simulink model "LACS"  (R2016b)
settings: Solver=VariableStepAuto  StartTime=0.0  StopTime=10  RelTol=1e-3
values from neighbouring files (symbols this model uses):
  coefficient = 0.8    [LACS.sldd]
  Detal_ref = 0.00022116955850615819 0.00022116955850615819 0.00024339323736781077 0.00026784369743330114 0.00029474273075037104 0.00032433393975435165 0.00035688482250496254 0.00039268904453642435 0.00043206891122917146 0.00047537805500027884 0.00052300435183202216 0.00057537308165349073 0.00063295034678974044 0.00069624676200566427 0.00076582142849131239 0.0008422862023284908 0.000926310265386283 0.0010186250    [LACS.sldd]    (also in path_generate.m = zeros(N,1))
  driver_decel = 4.0    [LACS.sldd]
  EgoLength = 3.048    [LACS.sldd]
  egopath = 0.0 0.25 0.5 0.75 1.0 1.25 1.5 1.7500000000000002 2.0 2.25 2.5 2.75 3.0 3.25 3.5000000000000004 3.75 4.0 4.25 4.5 4.75 5.0 5.25 5.5 5.75 6.0 6.25 6.5 6.75 7.0000000000000009 7.2499999999999991 7.5 7.75 8.0 8.25 8.5 8.75 9.0 9.25 9.5 9.75 10.0 10.25 10.5 10.75 11.0 11.25 11.5 11.75 12.0 12.25 12.5 12.75 13.0 13.25 13.5 13.750000000000002 14.000000000000002 14.250000000000002 14.499999999999998 14.7    [LACS.sldd]
  egoSpdLimit_H = 150.0    [LACS.sldd]
  egoSpdLimit_L = 10.0    [LACS.sldd]
  EgoWidth = 1.628    [LACS.sldd]
  ESA_Active = 3.0    [LACS.sldd]
  ESA_mask_1 = 31.0    [LACS.sldd]
  ESA_mask_2 = 15.0    [LACS.sldd]
  ESA_mask_3 = 255.0    [LACS.sldd]
  ESA_mask_4 = 31.0    [LACS.sldd]
  ESA_Passive = 1.0    [LACS.sldd]
  ESA_Standby = 2.0    [LACS.sldd]
  g = 9.8    [LACS.sldd]
  headwayoffset = 1.524    [LACS.sldd]
  LatAccelThershold = 0.05    [LACS.sldd]
  LatDis = 0.5    [LACS.sldd]
  LatSafetyThershold = 0.5    [LACS.sldd]
  LengthObj = 3.0    [LACS.sldd]
  ObjWidth = 2.0    [LACS.sldd]
  PB1_decel = 3.0    [LACS.sldd]
  PB2_decel = 5.0    [LACS.sldd]
  PB3_decel = 8.0    [LACS.sldd]
  Phi_dot_ref = 0.00085065224568106894 0.00085065224568106894 0.000936127966106986 0.0010301682404378703 0.0011336261186052523 0.0012474385378394444 0.001372634343205976 0.0015103430260158721 0.001661804233646022 0.0018283781058153412 0.0020115564932359636 0.0022129751145658549 0.0024344267064660809 0.0026778752189651235 0.0029454711038487576 0.0032395677369184911 0.0035627390050890382 0.0039177980756855638 0.004    [LACS.sldd]    (also in path_generate.m = zeros(N,1))
  Phi_ref = 0.00038406250525431664 0.00042271073336932769 0.00046524334565338114 0.00051204974395873044 0.000563558155980624 0.00062023946191088657 0.00068261138880285879 0.00075124310596315759 0.0008267602572639512 0.0009098504689462523 0.0010012693742370194 0.0011018471988988175 0.0012124959546271103 0.0013342172899504143 0.0014681110508986705 0.0016153846060911084 0.0017773629929370329 0.001955499943191484    [LACS.sldd]    (also in path_generate.m = phi_ref)
  SteerAngleLimit = 20.0    [LACS.sldd]
  SteerAngleSpdLimit = 20.0    [LACS.sldd]
  StrAngSpdThershold = 0.05    [LACS.sldd]
  StrAngThershold = 0.0    [LACS.sldd]
  Time2React = 1.2    [LACS.sldd]
  timeMargin = 0.5    [LACS.sldd]
  TTCthreshold1 = 2.5    [LACS.sldd]
  TTCthreshold3 = 1.0    [LACS.sldd]
  X_dot_ref = 10.0 10.0 10.0 9.9999999999999947 10.0 10.0 10.0 10.0 10.0 10.0 10.0 10.0 10.0 10.0 10.0 10.000000000000018 10.0 10.0 10.0 10.0 10.0 10.0 10.0 10.0 10.0 10.0 10.0 10.0 10.0 10.0 10.0 10.0 10.0 10.0 10.0 10.0 10.0 10.0 10.0 10.0 10.0 10.0 10.0 10.0 10.0 10.0 10.0 10.0 10.0 10.0 10.0 10.0 10.0 10.0 10.0 10.0 10.0 10.0 10.0 10.0 10.0 10.0 10.0 9.9999999999999289 10.0 10.0 10.0 10.0 10.0 10.0 10.0 10.    [LACS.sldd]    (also in path_generate.m = zeros(N,1))
  X_ref = 0.05 0.55 1.05 1.55 2.05 2.55 3.05 3.55 4.05 4.55 5.05 5.55 6.05 6.55 7.05 7.55 8.05 8.55 9.05 9.55 10.05 10.55 11.05 11.55 12.05 12.55 13.05 13.55 14.05 14.55 15.05 15.55 16.05 16.55 17.05 17.55 18.05 18.55 19.05 19.55 20.05 20.55 21.05 21.55 22.05 22.55 23.05 23.55 24.05 24.55 25.05 25.55 26.05 26.55 27.05 27.55 28.05 28.55 29.05 29.55 30.05 30.55 31.05 31.55 32.05 32.55 33.05 33.55 34.05 34.55    [LACS.sldd]    (also in path_generate.m = X_phi')
  Y_dot_ref = 0.0044363771042237217 0.0044363771042237217 0.00488273213335339 0.0053739322979981 0.0059144698111347933 0.0065092840662692251 0.0071638055584438178 0.0078840039934084845 0.0086764409570179273 0.0095483275445279979 0.01050758737719603 0.011562925461771293 0.012723903376023141 0.014001021290828194 0.015405807364013962 0.016950915064438028 0.018650229002128878 0.020518979854070446 0.0225738689793052    [LACS.sldd]    (also in path_generate.m = zeros(N,1))
  Y_ref = 0.0020016327462461514 0.0022031718511841521 0.0024249907063953382 0.0026691273130630077 0.0029378239279629127 0.0032335474185196523 0.0035590116218331136 0.0039172018997553045 0.0043114020994257287 0.0047452241472766251 0.005222640524503025 0.0057480198933628265 0.0063261661664513911 0.0069623613352525482 0.0076624123997939579 0.008432702767994656 0.0092802485212165574 0.010212759971323001 0.01123    [LACS.sldd]    (also in path_generate.m = zeros(N,1))
undefined symbols (not defined in the file or in its folder): ADR_ADRCycleTime, ADR_SteeringYawrateThresh_p, AEB_mask1, aubr, CAEB_AccelPdlPosLimit, CAEB_AccelPdlPosSpdThreshold, CAEB_CalAEBLongVelObjLimit_mps, CAEB_CalAEBVMaxDec_kmph, ESA_AESACTIVE, ESA_ERROR, ESA_ESAFunctionOFF, ESA_ESAFunctionON, ESA_ESASwichOFF, ESA_ESS_DriverSteeringNumThreshold, ESA_ESSACTIVE, ESA_ForewardCollissionLevel2, ESA_ForewardCollissionLevel3, ESA_OFF, ESA_PASSIVE, ESA_PLAN_AES, ESA_PLAN_ESSLEFT, ESA_PLAN_ESSRIGHT, ESA_PLAN_FAILURE, ESA_PLAN_OFF, ESA_PLAN_STANDBY, ESA_PLAN_WAIT, ESA_SPEEDLIMITH6_p, ESA_SPEEDLIMITH7_p, ESA_SPEEDLIMITL6_p, ESA_SPEEDLIMITL7_p, ESA_STANDBY, ESA_StrAngSpdT6_p, FromAngle2Rad, Kp, magnitude, tablebr, TTCthreshold, vubr
libraries: simulink x15, Solver_SF x9, simulink_extras x1
(part 2 of 5)

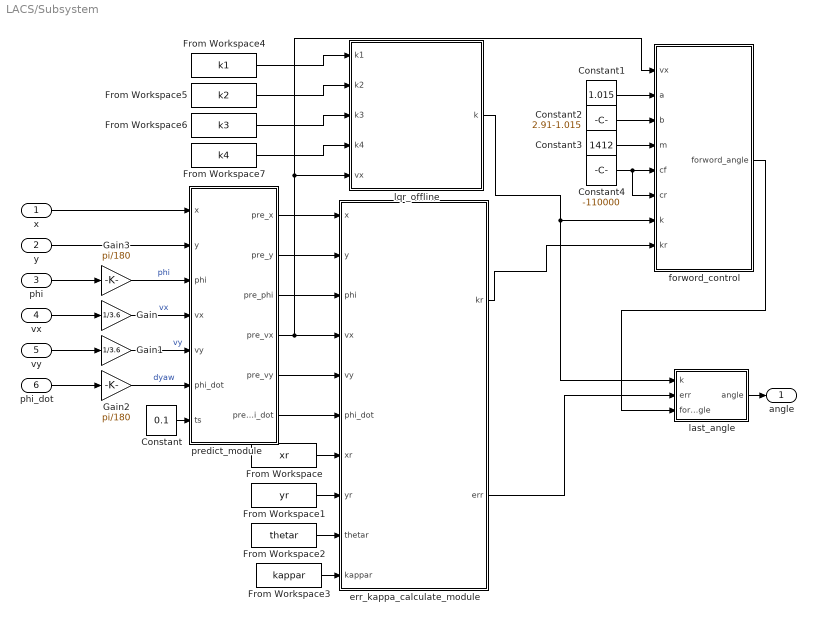
== system LACS/Subsystem ==
  x : Inport
  y : Inport  Port=2
  phi : Inport  Port=3
  vx : Inport  Port=4
  vy : Inport  Port=5
  phi_dot : Inport  Port=6
  Constant : Constant  Value=0.1
  Constant1 : Constant  Value=1.015
  Constant2 : Constant  Value=2.91-1.015
  Constant3 : Constant  Value=1412
  Constant4 : Constant  Value=-110000
  From Workspace : FromWorkspace  VariableName=xr  SampleTime=0
  From Workspace1 : FromWorkspace  VariableName=yr  SampleTime=0
  From Workspace2 : FromWorkspace  VariableName=thetar  SampleTime=0
  From Workspace3 : FromWorkspace  VariableName=kappar  SampleTime=0
  From Workspace4 : FromWorkspace  VariableName=k1  SampleTime=0
  From Workspace5 : FromWorkspace  VariableName=k2  SampleTime=0
  From Workspace6 : FromWorkspace  VariableName=k3  SampleTime=0
  From Workspace7 : FromWorkspace  VariableName=k4  SampleTime=0
  Gain : Gain  Gain=1/3.6
  Gain1 : Gain  Gain=1/3.6
  Gain2 : Gain  Gain=pi/180
  Gain3 : Gain  Gain=pi/180
  err_kappa_calculate_module : MATLAB Function  TreatAsAtomicUnit=on
  forword_control : MATLAB Function  TreatAsAtomicUnit=on
  last_angle : MATLAB Function  TreatAsAtomicUnit=on
  lqr_offline : MATLAB Function  TreatAsAtomicUnit=on
  predict_module : MATLAB Function  TreatAsAtomicUnit=on
  angle : Outport
  wires:
  From Workspace7/1 -> lqr_offline/4(k4)
  err_kappa_calculate_module/2(err) -> last_angle/2(err)
  Gain1/1 -> predict_module/5(vy)  "vy"
  From Workspace6/1 -> lqr_offline/3(k3)
  x/1 -> predict_module/1(x)
  lqr_offline/1(k) -> last_angle/1(k), forword_control/7(k)
  phi_dot/1 -> Gain2/1
  predict_module/2(pre_y) -> err_kappa_calculate_module/2(y)
  err_kappa_calculate_module/1(kr) -> forword_control/8(kr)
  forword_control/1(forword_angle) -> last_angle/3(forword_angle)
  vx/1 -> Gain/1
  predict_module/4(pre_vx) -> lqr_offline/5(vx), forword_control/1(vx), err_kappa_calculate_module/4(vx)
  Gain2/1 -> predict_module/6(phi_dot)  "dyaw"
  last_angle/1(angle) -> angle/1
  phi/1 -> Gain3/1
  From Workspace2/1 -> err_kappa_calculate_module/9(thetar)
  From Workspace5/1 -> lqr_offline/2(k2)
  Gain/1 -> predict_module/4(vx)  "vx"
  y/1 -> predict_module/2(y)
  Gain3/1 -> predict_module/3(phi)  "phi"
  From Workspace3/1 -> err_kappa_calculate_module/10(kappar)
  Constant/1 -> predict_module/7(ts)
  From Workspace4/1 -> lqr_offline/1(k1)
  From Workspace1/1 -> err_kappa_calculate_module/8(yr)
  predict_module/1(pre_x) -> err_kappa_calculate_module/1(x)
  predict_module/5(pre_vy) -> err_kappa_calculate_module/5(vy)
  vy/1 -> Gain1/1
  From Workspace/1 -> err_kappa_calculate_module/7(xr)
  predict_module/6(pre_phi_dot) -> err_kappa_calculate_module/6(phi_dot)
  predict_module/3(pre_phi) -> err_kappa_calculate_module/3(phi)
  Constant1/1 -> forword_control/2(a)
  Constant2/1 -> forword_control/3(b)
  Constant3/1 -> forword_control/4(m)
  Constant4/1 -> forword_control/6(cr), forword_control/5(cf)

== system LACS/TroqueOutput ==
  In1 : Inport
  Out1 : Outport

== system LACS/double_pid_controller ==
  s_dot : Inport
  v : Inport  Port=2
  es : Inport  Port=3
  rpm : Inport  Port=4
  vp : Inport  Port=5
  ap : Inport  Port=6
  Add : Sum  Inputs=-++
  Add2 : Sum
  Delay2 : Delay  DelayLength=1
  MATLAB Function1 : MATLAB Function  TreatAsAtomicUnit=on
  PID Controller : simulink/Continuous/PID Controller  Controller=PID  TimeDomain=Continuous-time  SampleTime=-1  IntegratorMethod=Forward Euler  FilterMethod=Forward Euler  Form=Parallel  UseFilter=on  ControllerParametersSource=internal  P=3  I=0  D=0.1  N=30  InitialConditionSource=internal  InitialConditionForIntegrator=0  InitialConditionForFilter=0  ExternalReset=none  LimitOutput=off  UpperSaturationLimit=inf  LowerSaturationLimit=-inf  LinearizeAsGain=on  AntiWindupMode=none  Kb=1  TrackingMode=off  Kt=1  PParamMin=[]  PParamMax=[]  IParamMin=[]  IParamMax=[]  DParamMin=[]  DParamMax=[]  NParamMin=[]  NParamMax=[]  KbParamMin=[]  KbParamMax=[]  KtParamMin=[]  KtParamMax=[]  POutMin=[]  POutMax=[]  IOutMin=[]  IOutMax=[]  DOutMin=[]  DOutMax=[]  NOutMin=[]  NOutMax=[]  KbOutMin=[]  KbOutMax=[]  KtOutMin=[]  KtOutMax=[]  IntegratorOutMin=[]  IntegratorOutMax=[]  FilterOutMin=[]  FilterOutMax=[]  SumOutMin=[]  SumOutMax=[]  SumI1OutMin=[]  SumI1OutMax=[]  SumI2OutMin=[]  SumI2OutMax=[]  SumI3OutMin=[]  SumI3OutMax=[]  SumDOutMin=[]  SumDOutMax=[]  SaturationOutMin=[]  SaturationOutMax=[]  IntegratorContinuousStateAttributes=''  IntegratorStateMustResolveToSignalObject=off  IntegratorRTWStateStorageClass=Auto  FilterContinuousStateAttributes=''  FilterStateMustResolveToSignalObject=off  FilterRTWStateStorageClass=Auto  DifferentiatorICPrevScaledInput=0  DifferentiatorOutMin=[]  DifferentiatorOutMax=[]
  PID Controller1 : simulink/Continuous/PID Controller  Controller=PID  TimeDomain=Continuous-time  SampleTime=-1  IntegratorMethod=Forward Euler  FilterMethod=Forward Euler  Form=Parallel  UseFilter=on  ControllerParametersSource=internal  P=3  I=0  D=0.1  N=30  InitialConditionSource=internal  InitialConditionForIntegrator=0  InitialConditionForFilter=0  ExternalReset=none  LimitOutput=off  UpperSaturationLimit=inf  LowerSaturationLimit=-inf  LinearizeAsGain=on  AntiWindupMode=none  Kb=1  TrackingMode=off  Kt=1  PParamMin=[]  PParamMax=[]  IParamMin=[]  IParamMax=[]  DParamMin=[]  DParamMax=[]  NParamMin=[]  NParamMax=[]  KbParamMin=[]  KbParamMax=[]  KtParamMin=[]  KtParamMax=[]  POutMin=[]  POutMax=[]  IOutMin=[]  IOutMax=[]  DOutMin=[]  DOutMax=[]  NOutMin=[]  NOutMax=[]  KbOutMin=[]  KbOutMax=[]  KtOutMin=[]  KtOutMax=[]  IntegratorOutMin=[]  IntegratorOutMax=[]  FilterOutMin=[]  FilterOutMax=[]  SumOutMin=[]  SumOutMax=[]  SumI1OutMin=[]  SumI1OutMax=[]  SumI2OutMin=[]  SumI2OutMax=[]  SumI3OutMin=[]  SumI3OutMax=[]  SumDOutMin=[]  SumDOutMax=[]  SaturationOutMin=[]  SaturationOutMax=[]  IntegratorContinuousStateAttributes=''  IntegratorStateMustResolveToSignalObject=off  IntegratorRTWStateStorageClass=Auto  FilterContinuousStateAttributes=''  FilterStateMustResolveToSignalObject=off  FilterRTWStateStorageClass=Auto  DifferentiatorICPrevScaledInput=0  DifferentiatorOutMin=[]  DifferentiatorOutMax=[]
  Saturation : Saturate  UpperLimit=5  LowerLimit=-8
  Saturation1 : Saturate  UpperLimit=10  LowerLimit=-10
  moto model : MATLAB Function  TreatAsAtomicUnit=on
  油门刹车合并标定表 : Lookup_n-D  BreakpointsForDimension1=vubr  BreakpointsForDimension2=aubr  Table=tablebr  InternalRulePriority=Speed  RndMeth=Simplest  InputSameDT=on
  Out1 : Outport
  Out2 : Outport  Port=2
  wires:
  v/1 -> Delay2/1
  ap/1 -> Add2/2
  Add2/1 -> Saturation/1
  Saturation/1 -> 油门刹车合并标定表/2
  Delay2/1 -> 油门刹车合并标定表/1
  油门刹车合并标定表/1 -> MATLAB Function1/1(x)
  Add/1 -> PID Controller/1
  PID Controller/1 -> Add2/1
  MATLAB Function1/1(thr) -> moto model/1(thr)
  PID Controller1/1 -> Saturation1/1
  moto model/1(torque) -> Out1/1
  MATLAB Function1/2(brake) -> Out2/1
  vp/1 -> Add/3
  es/1 -> PID Controller1/1
  s_dot/1 -> Add/1
  rpm/1 -> moto model/2(rpm)
  Saturation1/1 -> Add/2

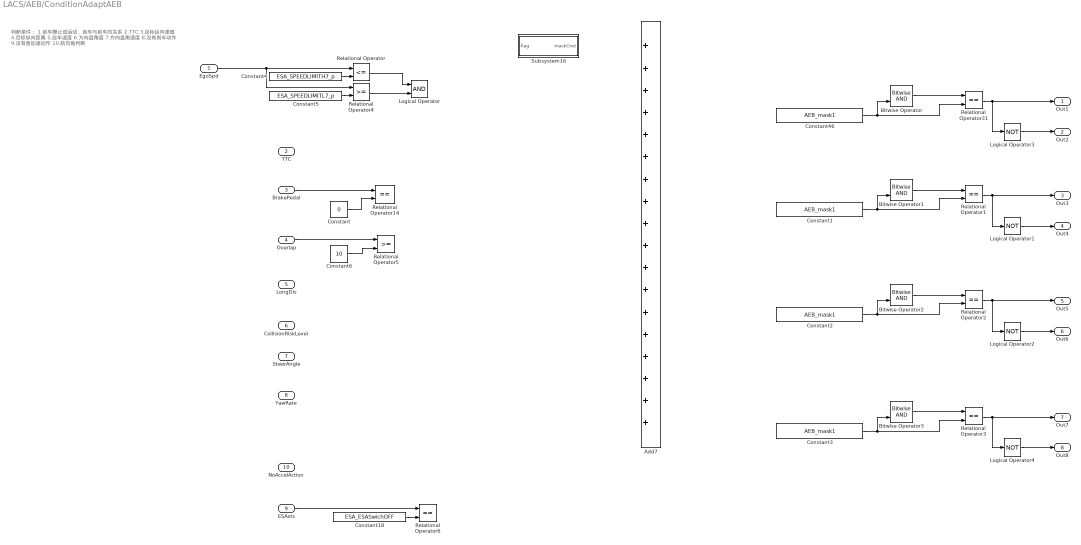
== system LACS/AEB/ConditionAdaptAEB ==
  note: 判断条件：
      | 1.前车静止或运动，自车与前车的关系
      | 2.TTC
      | 3.目标纵向速度
      | 4.目标纵向距离
      | 5.自车速度
      | 6.方向盘角度
      | 7.方向盘角速度
      | 8.没有刹车动作
      | 9.没有急加速动作
      | 10.航向角判断
  EgoSpd : Inport
  TTC : Inport  Port=2
  BrakePedal : Inport  Port=3
  Overlap : Inport  Port=4
  LongDis : Inport  Port=5
  CollisionRiskLevel : Inport  Port=6
  SteerAngle : Inport  Port=7
  YawRate : Inport  Port=8
  ESAsts : Inport  Port=9
  NoAccelAction : Inport  Port=10
  Add7 : Sum  Inputs=18  SaturateOnIntegerOverflow=on
  Bitwise Operator{,1..3} (4 alike) : simulink/Logic and Bit Operations/Bitwise Operator  logicop=AND  UseBitMask=off  NumInputPorts=2  BitMask=bin2dec('11011001')  BitMaskRealWorld=Stored Integer
  Constant : Constant  Value=0
  Constant{1..3,46} (4 alike) : Constant  Value=AEB_mask1  OutDataTypeStr=uint32
  Constant18 : Constant  Value=ESA_ESASwichOFF
  Constant4 : Constant  Value=ESA_SPEEDLIMITH7_p
  Constant5 : Constant  Value=ESA_SPEEDLIMITL7_p
  Constant6 : Constant  Value=10
  Logical Operator : Logic  AllPortsSameDT=off  OutDataTypeStr=boolean
  Logical Operator{1..4} (4 alike) : Logic  Operator=NOT  AllPortsSameDT=off  OutDataTypeStr=boolean
  Relational Operator : RelationalOperator  Operator=<=  OutDataTypeStr=boolean  RndMeth=Simplest
  Relational Operator{1..3,6,14,31} (6 alike) : RelationalOperator  Operator===  OutDataTypeStr=boolean  RndMeth=Simplest
  Relational Operator4 : RelationalOperator  OutDataTypeStr=boolean  RndMeth=Simplest
  Relational Operator5 : RelationalOperator  OutDataTypeStr=boolean  RndMeth=Simplest
  Subsystem16 : Subsystem
  Out1 : Outport
  Out2 : Outport  Port=2
  Out3 : Outport  Port=3
  Out4 : Outport  Port=4
  Out5 : Outport  Port=5
  Out6 : Outport  Port=6
  Out7 : Outport  Port=7
  Out8 : Outport  Port=8
  wires:
  Constant46/1 -> Bitwise Operator/2, Relational Operator31/2
  Bitwise Operator/1 -> Relational Operator31/1
  Relational Operator31/1 -> Logical Operator3/1, Out1/1
  Logical Operator3/1 -> Out2/1
  Constant1/1 -> Bitwise Operator1/2, Relational Operator1/2
  Bitwise Operator1/1 -> Relational Operator1/1
  Relational Operator1/1 -> Logical Operator1/1, Out3/1
  Logical Operator1/1 -> Out4/1
  Constant2/1 -> Bitwise Operator2/2, Relational Operator2/2
  Bitwise Operator2/1 -> Relational Operator2/1
  Relational Operator2/1 -> Logical Operator2/1, Out5/1
  Logical Operator2/1 -> Out6/1
  Constant3/1 -> Bitwise Operator3/2, Relational Operator3/2
  Bitwise Operator3/1 -> Relational Operator3/1
  Relational Operator3/1 -> Logical Operator4/1, Out7/1
  Logical Operator4/1 -> Out8/1
  Constant/1 -> Relational Operator14/2
  BrakePedal/1 -> Relational Operator14/1
  Relational Operator/1 -> Logical Operator/1
  Relational Operator4/1 -> Logical Operator/2
  EgoSpd/1 -> Relational Operator/1, Relational Operator4/1
  Constant4/1 -> Relational Operator/2
  Constant5/1 -> Relational Operator4/2
  Constant6/1 -> Relational Operator5/2
  Overlap/1 -> Relational Operator5/1
  ESAsts/1 -> Relational Operator6/1
  Constant18/1 -> Relational Operator6/2

== system LACS/AEB/DrvRapidAccelAction ==
  AccelPedalPos : Inport
  Add : Sum  Inputs=+-
  CAEB_AccelPdlPosLimit : Constant  Value=CAEB_AccelPdlPosLimit  OutDataTypeStr=Inherit: Inherit via back propagation
  CAEB_IPBInputRodStrokeSpdThreshold : Constant  Value=CAEB_AccelPdlPosSpdThreshold  OutDataTypeStr=single
  Constant4 : Constant  Value=0.02  OutDataTypeStr=single
  Data Type Conversion : DataTypeConversion
  Delay : Delay  DelayLength=1
  Divide : Product  Inputs=*//
  Logical Operator : Logic  AllPortsSameDT=off  OutDataTypeStr=boolean
  Relational Operator17 : RelationalOperator  OutDataTypeStr=boolean  RndMeth=Simplest
  Relational Operator4 : RelationalOperator  OutDataTypeStr=boolean  RndMeth=Simplest
  Saturation : Saturate  UpperLimit=inf  LowerLimit=0.0001
  DrvRapidAccelAction : Outport
  wires:
  CAEB_AccelPdlPosLimit/1 -> Relational Operator17/2
  Delay/1 -> Add/2
  Add/1 -> Divide/1
  AccelPedalPos/1 -> Data Type Conversion/1, Delay/1, Add/1, Relational Operator17/1
  Data Type Conversion/1 -> Saturation/1
  Saturation/1 -> Divide/2
  Constant4/1 -> Divide/3
  Divide/1 -> Relational Operator4/1
  CAEB_IPBInputRodStrokeSpdThreshold/1 -> Relational Operator4/2
  Relational Operator17/1 -> Logical Operator/1
  Relational Operator4/1 -> Logical Operator/2
  Logical Operator/1 -> DrvRapidAccelAction/1

== system LACS/AEB/TTCCaculation ==
  LongiVel : Inport
  LongiDis : Inport  Port=2
  Abs : Abs
  Abs1 : Abs
  Divide : Product  Inputs=*/
  Saturation1 : Saturate  UpperLimit=inf  LowerLimit=CAEB_CalAEBLongVelObjLimit_mps
  Saturation2 : Saturate  UpperLimit=inf  LowerLimit=CAEB_CalAEBLongVelObjLimit_mps
  TTC : Outport
  wires:
  LongiVel/1 -> Abs/1
  Abs/1 -> Saturation1/1
  LongiDis/1 -> Saturation2/1
  Abs1/1 -> TTC/1
  Divide/1 -> Abs1/1
  Saturation2/1 -> Divide/1
  Saturation1/1 -> Divide/2

== system LACS/AEB//ESAModeSwitch/If Action Subsystem ==
  Action Port : ActionPort  ActionType=then
  Constant1 : Constant  OutDataTypeStr=boolean
  Constant2 : Constant  Value=0  OutDataTypeStr=boolean
  ESAVTakeOverReq : Outport
  AEBVCrashAvoid : Outport  Port=2
  wires:
  Constant1/1 -> ESAVTakeOverReq/1
  Constant2/1 -> AEBVCrashAvoid/1

== system LACS/AEB//ESAModeSwitch/If Action Subsystem1 ==
  AEBTTCVaild : Inport
  EgoSpd : Inport  Port=2
  AEBTTC : Inport  Port=3
  Action Port : ActionPort  ActionType=else
  If : If  IfExpression=u1==0|u1==1|u1==4  ElseIfExpressions=u1==2
  If Action Subsystem : Subsystem  TreatAsAtomicUnit=on
  If Action Subsystem1 : Subsystem  TreatAsAtomicUnit=on
  If Action Subsystem2 : Subsystem  TreatAsAtomicUnit=on
  Merge : Merge  Inputs=3
  Merge1 : Merge  Inputs=3
  ESAVTakeOverReq : Outport
  AEBVCrashAvoid : Outport  Port=2
  wires:
  If/1 -> If Action Subsystem/Action
  If/2 -> If Action Subsystem1/Action
  If/3 -> If Action Subsystem2/Action
  Merge/1 -> ESAVTakeOverReq/1
  If Action Subsystem/1(ESAVTakeOverReq) -> Merge/1
  If Action Subsystem1/1(ESAVTakeOverReq) -> Merge/2
  If Action Subsystem2/1(ESAVTakeOverReq) -> Merge/3
  If Action Subsystem1/2(AEBVCrashAvoid) -> Merge1/2
  Merge1/1 -> AEBVCrashAvoid/1
  If Action Subsystem/2(AEBVCrashAvoid) -> Merge1/1
  If Action Subsystem2/2(AEBVCrashAvoid) -> Merge1/3
  AEBTTCVaild/1 -> If Action Subsystem/1(AEBTTCVaild), If/1
  AEBTTC/1 -> If Action Subsystem/2(AEBTTC), If Action Subsystem1/1(AEBTTC)
  EgoSpd/1 -> If Action Subsystem/3(EgoSpd), If Action Subsystem1/2(EgoSpd)

== system LACS/AEB//ESAModeSwitch/Subsystem ==
  SteerAngle : Inport
  SteerAngleSpd : Inport  Port=2
  Abs : Abs
  Abs1 : Abs
  Add1 : Sum  SaturateOnIntegerOverflow=on
  Add3 : Sum  SaturateOnIntegerOverflow=on
  Constant1 : Constant  Value=ESA_SPEEDLIMITH6_p
  Constant17 : Constant  OutDataTypeStr=uint8
  Constant18 : Constant  Value=0  OutDataTypeStr=uint8
  Constant2 : Constant  Value=ESA_SPEEDLIMITH6_p
  Constant22 : Constant  Value=ESA_StrAngSpdT6_p
  Constant3 : Constant  OutDataTypeStr=uint8
  Constant4 : Constant  Value=0  OutDataTypeStr=uint8
  Constant5 : Constant  Value=ESA_StrAngSpdT6_p
  Logical Operator : Logic  AllPortsSameDT=off  OutDataTypeStr=boolean
  Multiport Switch1 : MultiPortSwitch  DataPortOrder=Zero-based contiguous  Inputs=2
  Multiport Switch2 : MultiPortSwitch  DataPortOrder=Zero-based contiguous  Inputs=2
  Relational Operator{1..3,19} (4 alike) : RelationalOperator  OutDataTypeStr=boolean  RndMeth=Simplest
  Unit Delay1 : UnitDelay  SampleTime=-1
  Unit Delay2 : UnitDelay  SampleTime=-1
  DrvRapidSteerAction : Outport
  wires:
  Abs/1 -> Relational Operator2/1
  Relational Operator19/1 -> Logical Operator/1
  Constant1/1 -> Relational Operator1/2
  Abs1/1 -> Relational Operator1/1
  SteerAngleSpd/1 -> Abs1/1
  Logical Operator/1 -> DrvRapidSteerAction/1
  Multiport Switch2/1 -> Relational Operator19/1, Unit Delay2/1
  Constant2/1 -> Relational Operator2/2
  SteerAngle/1 -> Abs/1
  Constant18/1 -> Multiport Switch2/2
  Relational Operator2/1 -> Multiport Switch2/1
  Add3/1 -> Multiport Switch2/3
  Constant22/1 -> Relational Operator19/2
  Constant17/1 -> Add3/1
  Unit Delay2/1 -> Add3/2
  Relational Operator3/1 -> Logical Operator/2
  Constant4/1 -> Multiport Switch1/2
  Relational Operator1/1 -> Multiport Switch1/1
  Constant3/1 -> Add1/1
  Add1/1 -> Multiport Switch1/3
  Unit Delay1/1 -> Add1/2
  Constant5/1 -> Relational Operator3/2
  Multiport Switch1/1 -> Relational Operator3/1, Unit Delay1/1

== system LACS/AEBsts/Brake2StopTime ==
  EgoSpd : Inport
  CMpa1 : Inport  Port=2
  CMpa2 : Inport  Port=3
  CMpa3 : Inport  Port=4
  Add{1..4} (4 alike) : Sum
  Constant : Constant  Value=driver_decel
  Constant1 : Constant  Value=timeMargin
  Constant2 : Constant  Value=Time2React
  Divide{,1..3} (4 alike) : Product  Inputs=*/
  FCWStoppingTime : Outport
  PB1StoppingTime : Outport  Port=2
  PB2StoppingTime : Outport  Port=3
  FBStoppingTime : Outport  Port=4
  tag scope: FBStoppingTime=global, FCWStopTime_M=global, PB1StoppingTime_M=global, PB2StoppingTime_M=global
  wires:
  Constant/1 -> Divide/2
  EgoSpd/1 -> Divide1/1, Divide3/1, Divide2/1, Divide/1
  Constant2/1 -> Add1/1
  Divide/1 -> Add1/2
  Add1/1 -> [FCWStopTime_M], FCWStoppingTime/1
  Constant1/1 -> Add4/1, Add3/1, Add2/1
  Divide1/1 -> Add2/2
  CMpa2/1 -> Divide2/2
  Divide2/1 -> Add3/2
  Add3/1 -> [PB2StoppingTime_M], PB2StoppingTime/1
  CMpa3/1 -> Divide3/2
  Divide3/1 -> Add4/2
  Add4/1 -> [FBStoppingTime], FBStoppingTime/1
  Add2/1 -> [PB1StoppingTime_M], PB1StoppingTime/1
  CMpa1/1 -> Divide1/2

== system LACS/AEBsts/TTCCaculation ==
  LongiDis : Inport
  LongiVel : Inport  Port=2
  Abs : Abs
  Abs1 : Abs
  Add : Sum  Inputs=+-
  Constant : Constant  Value=headwayoffset
  Constant1 : Constant  Value=0.1
  Divide : Product  Inputs=*/
  Relational Operator4 : RelationalOperator  Operator=<  OutDataTypeStr=boolean  RndMeth=Simplest
  collision : Outport
  TTC : Outport  Port=2
  tag scope: LongiDis_M=global, Longivel_M=global, TTC_M=global, collision_M=global
  wires:
  LongiVel/1 -> Abs/1
  Abs/1 -> [Longivel_M], Divide/2
  LongiDis/1 -> [LongiDis_M], Add/1
  Add/1 -> Relational Operator4/1, Divide/1
  Constant/1 -> Add/2
  Constant1/1 -> Relational Operator4/2
  Relational Operator4/1 -> [collision_M], collision/1
  Divide/1 -> Abs1/1
  Abs1/1 -> [TTC_M], TTC/1

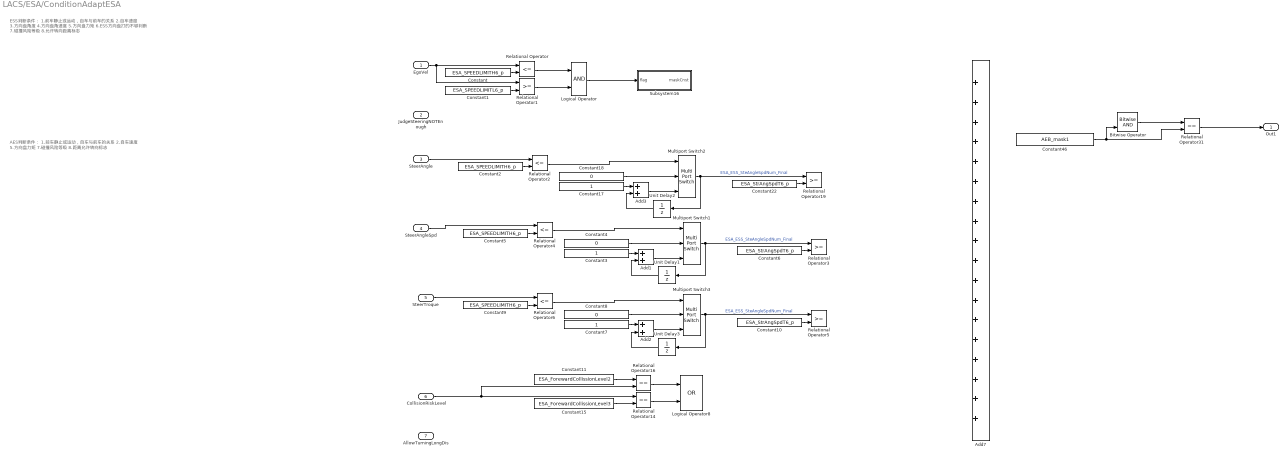
== system LACS/ESA/ConditionAdaptESA ==
  note: ESS判断条件：
      | 1.前车静止或运动，自车与前车的关系
      | 2.自车速度
      | 3.方向盘角度
      | 4.方向盘角速度
      | 5.方向盘力矩
      | 6.ESS方向盘打的不够判断
      | 7.碰撞风险等级
      | 8.允许转向距离标志
  note: AES判断条件：
      | 1.前车静止或运动，自车与前车的关系
      | 2.自车速度
      | 5.方向盘力矩
      | 7.碰撞风险等级
      | 8.距离允许转向标志
  EgoVel : Inport
  JudgeSteeringNOTEnough : Inport  Port=2
  SteerAngle : Inport  Port=3
  SteerAngleSpd : Inport  Port=4
  SteerTroque : Inport  Port=5
  CollisionRiskLevel : Inport  Port=6
  AllowTurningLongDis : Inport  Port=7
  Add1 : Sum  SaturateOnIntegerOverflow=on
  Add2 : Sum  SaturateOnIntegerOverflow=on
  Add3 : Sum  SaturateOnIntegerOverflow=on
  Add7 : Sum  Inputs=18  SaturateOnIntegerOverflow=on
  Bitwise Operator : simulink/Logic and Bit Operations/Bitwise Operator  logicop=AND  UseBitMask=off  NumInputPorts=2  BitMask=bin2dec('11011001')  BitMaskRealWorld=Stored Integer
  Constant{,2,5,9} (4 alike) : Constant  Value=ESA_SPEEDLIMITH6_p
  Constant1 : Constant  Value=ESA_SPEEDLIMITL6_p
  Constant10 : Constant  Value=ESA_StrAngSpdT6_p
  Constant11 : Constant  Value=ESA_ForewardCollissionLevel2  OutDataTypeStr=uint8
  Constant15 : Constant  Value=ESA_ForewardCollissionLevel3  OutDataTypeStr=uint8
  Constant17 : Constant  OutDataTypeStr=uint8
  Constant18 : Constant  Value=0  OutDataTypeStr=uint8
  Constant22 : Constant  Value=ESA_StrAngSpdT6_p
  Constant3 : Constant  OutDataTypeStr=uint8
  Constant4 : Constant  Value=0  OutDataTypeStr=uint8
  Constant46 : Constant  Value=AEB_mask1  OutDataTypeStr=uint32
  Constant6 : Constant  Value=ESA_StrAngSpdT6_p
  Constant7 : Constant  OutDataTypeStr=uint8
  Constant8 : Constant  Value=0  OutDataTypeStr=uint8
  Logical Operator : Logic  AllPortsSameDT=off  OutDataTypeStr=boolean
  Logical Operator8 : Logic  Operator=OR  AllPortsSameDT=off  OutDataTypeStr=boolean
  Multiport Switch1 : MultiPortSwitch  DataPortOrder=Zero-based contiguous  Inputs=2
  Multiport Switch2 : MultiPortSwitch  DataPortOrder=Zero-based contiguous  Inputs=2
  Multiport Switch3 : MultiPortSwitch  DataPortOrder=Zero-based contiguous  Inputs=2
  Relational Operator{,2,4,6} (4 alike) : RelationalOperator  Operator=<=  OutDataTypeStr=boolean  RndMeth=Simplest
  Relational Operator{1,3,5,19} (4 alike) : RelationalOperator  OutDataTypeStr=boolean  RndMeth=Simplest
  Relational Operator14 : RelationalOperator  Operator===  OutDataTypeStr=boolean  RndMeth=Simplest
  Relational Operator16 : RelationalOperator  Operator===  OutDataTypeStr=boolean  RndMeth=Simplest
  Relational Operator31 : RelationalOperator  Operator===  OutDataTypeStr=boolean  RndMeth=Simplest
  Subsystem16 : Subsystem
  Unit Delay1 : UnitDelay  SampleTime=-1
  Unit Delay2 : UnitDelay  SampleTime=-1
  Unit Delay3 : UnitDelay  SampleTime=-1
  Out1 : Outport
  wires:
  Constant46/1 -> Bitwise Operator/2, Relational Operator31/2
  Bitwise Operator/1 -> Relational Operator31/1
  Relational Operator31/1 -> Out1/1
  Constant1/1 -> Relational Operator1/2
  Constant/1 -> Relational Operator/2
  EgoVel/1 -> Relational Operator/1, Relational Operator1/1
  Relational Operator1/1 -> Logical Operator/2
  Relational Operator/1 -> Logical Operator/1
  Logical Operator/1 -> Subsystem16/1(flag)
  Constant2/1 -> Relational Operator2/2
  SteerAngle/1 -> Relational Operator2/1
  Add3/1 -> Multiport Switch2/3
  Constant17/1 -> Add3/1
  Unit Delay2/1 -> Add3/2
  Constant22/1 -> Relational Operator19/2
  Multiport Switch2/1 -> Unit Delay2/1, Relational Operator19/1  "ESA_ESS_SteAngleSpdNum_Final"
  Constant18/1 -> Multiport Switch2/2
  Relational Operator2/1 -> Multiport Switch2/1
  Constant5/1 -> Relational Operator4/2
  SteerAngleSpd/1 -> Relational Operator4/1
  Add1/1 -> Multiport Switch1/3
  Constant3/1 -> Add1/1
  Unit Delay1/1 -> Add1/2
  Constant6/1 -> Relational Operator3/2
  Multiport Switch1/1 -> Unit Delay1/1, Relational Operator3/1  "ESA_ESS_SteAngleSpdNum_Final"
  Constant4/1 -> Multiport Switch1/2
  Relational Operator4/1 -> Multiport Switch1/1
  Constant9/1 -> Relational Operator6/2
  SteerTroque/1 -> Relational Operator6/1
  Add2/1 -> Multiport Switch3/3
  Constant7/1 -> Add2/1
  Unit Delay3/1 -> Add2/2
  Constant10/1 -> Relational Operator5/2
  Multiport Switch3/1 -> Unit Delay3/1, Relational Operator5/1  "ESA_ESS_SteAngleSpdNum_Final"
  Constant8/1 -> Multiport Switch3/2
  Relational Operator6/1 -> Multiport Switch3/1
  Constant15/1 -> Relational Operator14/2
  CollisionRiskLevel/1 -> Relational Operator16/2, Relational Operator14/1
  Constant11/1 -> Relational Operator16/1
  Relational Operator16/1 -> Logical Operator8/1
  Relational Operator14/1 -> Logical Operator8/2

== system LACS/ESA/Control ==
  In1 : Inport
  Out1 : Outport

== system LACS/ESA/OverlapCaculation ==
  LatSpd : Inport
  TTC : Inport  Port=2
  LatDis : Inport  Port=3
  VehicleWidth : Inport  Port=4
  Abs : Abs
  Add5 : Sum
  Add6 : Sum  Inputs=+-
  Constant1 : Constant  Value=100
  Constant2 : Constant  Value=100
  Constant3 : Constant  Value=0.5
  Divide : Product  Inputs=*/
  Product1 : Product
  Product2 : Product
  Product3 : Product
  Saturation1 : Saturate  UpperLimit=20  LowerLimit=-20
  Saturation2 : Saturate  UpperLimit=100  LowerLimit=0
  OverLap : Outport
  wires:
  LatSpd/1 -> Product1/1
  TTC/1 -> Product1/2
  Constant2/1 -> Product2/1
  Divide/1 -> Product2/2
  VehicleWidth/1 -> Product3/1
  Saturation2/1 -> Add6/2
  Constant1/1 -> Add6/1
  LatDis/1 -> Add5/2
  Add6/1 -> OverLap/1
  Add5/1 -> Saturation1/1
  Product1/1 -> Add5/1
  Product2/1 -> Saturation2/1
  Product3/1 -> Divide/2
  Constant3/1 -> Product3/2
  Abs/1 -> Divide/1
  Saturation1/1 -> Abs/1

== system LACS/ESA/SteerDirection ==
  note: ESAsts=ESS
  ESAsts : Inport
  YawRate : Inport  Port=2
  FixSelectObs : Inport  Port=3
  Constant : Constant  Value=0
  Constant1 : Constant  Value=0
  If : If  IfExpression=u1 == 3  ElseIfExpressions=u1 == 4
  If Action Subsystem1 : Subsystem  TreatAsAtomicUnit=on
  Logical Operator : Logic  AllPortsSameDT=off  OutDataTypeStr=boolean
  Logical Operator1 : Logic  AllPortsSameDT=off  OutDataTypeStr=boolean
  Relational Operator : RelationalOperator  Operator=>  OutDataTypeStr=boolean  RndMeth=Simplest
  Relational Operator1 : RelationalOperator  Operator=<  OutDataTypeStr=boolean  RndMeth=Simplest
  Subsystem : Subsystem
  Subsystem1 : Subsystem
  ESS_LeftCtrl : Outport
  ESS_RightCtrl : Outport  Port=2
  CtrlInvaild : Outport  Port=3
  AES_LeftCtrl : Outport  Port=4
  AES_RightCtrl : Outport  Port=5
  wires:
  ESAsts/1 -> If/1
  If/1 -> Subsystem/Action
  If/3 -> If Action Subsystem1/Action
  Subsystem/1(Out2) -> Logical Operator1/1, Logical Operator/1
  Constant/1 -> Relational Operator/2
  Relational Operator/1 -> Logical Operator/2
  YawRate/1 -> Relational Operator1/1, Relational Operator/1, Subsystem/1(In1)
  Constant1/1 -> Relational Operator1/2
  Relational Operator1/1 -> Logical Operator1/2
  If Action Subsystem1/1(Out1) -> CtrlInvaild/1
  Logical Operator/1 -> ESS_LeftCtrl/1
  Logical Operator1/1 -> ESS_RightCtrl/1
  If/2 -> Subsystem1/Action
  FixSelectObs/1 -> Subsystem1/1(In1)
  Subsystem1/1(Left) -> AES_LeftCtrl/1
  Subsystem1/2(Right) -> AES_RightCtrl/1

== system LACS/ESA/TrajactoryPlan ==
  EgoSpd : Inport
  YawRate : Inport  Port=2
  Abs : Abs
  Constant : Constant  Value=ADR_SteeringYawrateThresh_p  OutDataTypeStr=single
  Constant1 : Constant  Value=FromAngle2Rad
  Multiport Switch : MultiPortSwitch  DataPortOrder=Zero-based contiguous  Inputs=2
  Product : Product  Inputs=**
  Relational Operator : RelationalOperator  Operator=<=  OutDataTypeStr=boolean  RndMeth=Simplest
  Steering : Subsystem
  Straight : Subsystem
  Pos_ego : Outport
  wires:
  Multiport Switch/1 -> Pos_ego/1
  Constant1/1 -> Product/2
  Product/1 -> Abs/1, Steering/1(yawrate)
  Straight/1(dPos_ego) -> Multiport Switch/3
  Steering/1(dPos_ego) -> Multiport Switch/2
  Relational Operator/1 -> Multiport Switch/1
  Constant/1 -> Relational Operator/2
  Abs/1 -> Relational Operator/1
  EgoSpd/1 -> Straight/1(velocity), Steering/2(velocity)
  YawRate/1 -> Product/1

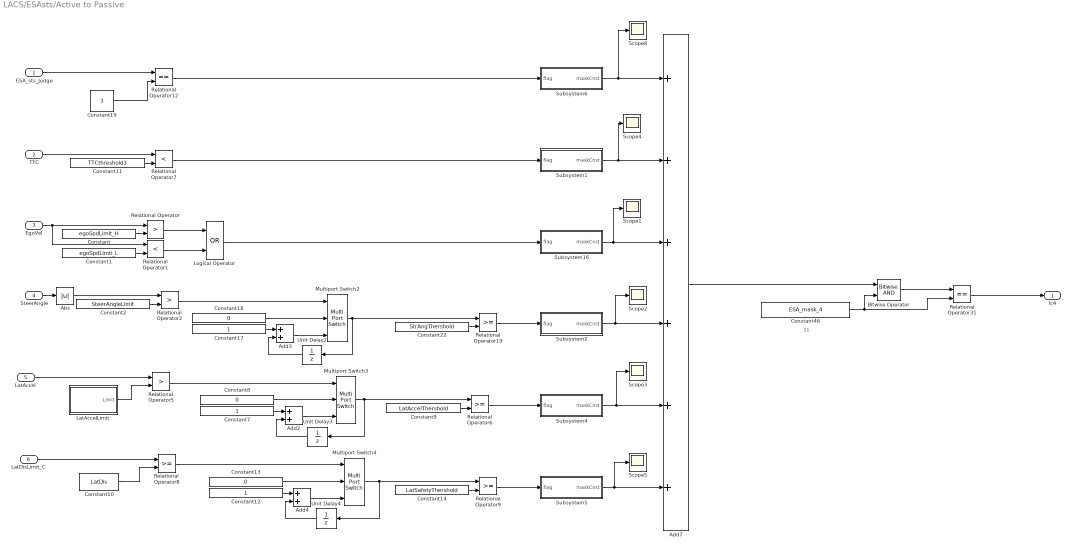
== system LACS/ESAsts/Active to Passive ==
  note: 31
  ESA_sts_Judge : Inport
  TTC : Inport  Port=2
  EgoVel : Inport  Port=3
  SteerAngle : Inport  Port=4
  LatAccel : Inport  Port=5
  LatDisLimit_C : Inport  Port=6
  Abs : Abs
  Add2 : Sum  SaturateOnIntegerOverflow=on
  Add3 : Sum  SaturateOnIntegerOverflow=on
  Add4 : Sum  SaturateOnIntegerOverflow=on
  Add7 : Sum  Inputs=6  SaturateOnIntegerOverflow=on
  Bitwise Operator : simulink/Logic and Bit Operations/Bitwise Operator  logicop=AND  UseBitMask=off  NumInputPorts=2  BitMask=bin2dec('11011001')  BitMaskRealWorld=Stored Integer
  Constant : Constant  Value=egoSpdLimit_H
  Constant1 : Constant  Value=egoSpdLimit_L
  Constant10 : Constant  Value=LatDis
  Constant11 : Constant  Value=TTCthreshold3
  Constant12 : Constant  OutDataTypeStr=uint8
  Constant13 : Constant  Value=0  OutDataTypeStr=uint8
  Constant14 : Constant  Value=LatSafetyThershold
  Constant17 : Constant  OutDataTypeStr=uint8
  Constant18 : Constant  Value=0  OutDataTypeStr=uint8
  Constant19 : Constant  Value=3
  Constant2 : Constant  Value=SteerAngleLimit
  Constant22 : Constant  Value=StrAngThershold
  Constant46 : Constant  Value=ESA_mask_4  OutDataTypeStr=uint32
  Constant7 : Constant  OutDataTypeStr=uint8
  Constant8 : Constant  Value=0  OutDataTypeStr=uint8
  Constant9 : Constant  Value=LatAccelThershold
  LatAccelLimit : Subsystem
  Logical Operator : Logic  Operator=OR  AllPortsSameDT=off  OutDataTypeStr=boolean
  Multiport Switch2 : MultiPortSwitch  DataPortOrder=Zero-based contiguous  Inputs=2
  Multiport Switch3 : MultiPortSwitch  DataPortOrder=Zero-based contiguous  Inputs=2
  Multiport Switch4 : MultiPortSwitch  DataPortOrder=Zero-based contiguous  Inputs=2
  Relational Operator : RelationalOperator  Operator=>  OutDataTypeStr=boolean  RndMeth=Simplest
  Relational Operator1 : RelationalOperator  Operator=<  OutDataTypeStr=boolean  RndMeth=Simplest
  Relational Operator12 : RelationalOperator  Operator===  OutDataTypeStr=boolean  RndMeth=Simplest
  Relational Operator{6,8..9,19} (4 alike) : RelationalOperator  OutDataTypeStr=boolean  RndMeth=Simplest
  Relational Operator2 : RelationalOperator  Operator=>  OutDataTypeStr=boolean  RndMeth=Simplest
  Relational Operator31 : RelationalOperator  Operator===  OutDataTypeStr=boolean  RndMeth=Simplest
  Relational Operator5 : RelationalOperator  Operator=>  OutDataTypeStr=boolean  RndMeth=Simplest
  Relational Operator7 : RelationalOperator  Operator=<  OutDataTypeStr=boolean  RndMeth=Simplest
  Scope{1..5,8} (6 alike) : Scope
  Subsystem1 : Subsystem
  Subsystem16 : Subsystem
  Subsystem2 : Subsystem
  Subsystem4 : Subsystem
  Subsystem5 : Subsystem
  Subsystem6 : Subsystem
  Unit Delay2 : UnitDelay  SampleTime=-1
  Unit Delay3 : UnitDelay  SampleTime=-1
  Unit Delay4 : UnitDelay  SampleTime=-1
  fc4 : Outport
  wires:
  Constant46/1 -> Bitwise Operator/2, Relational Operator31/2
  Bitwise Operator/1 -> Relational Operator31/1
  Relational Operator31/1 -> fc4/1
  Constant1/1 -> Relational Operator1/2
  Constant/1 -> Relational Operator/2
  EgoVel/1 -> Relational Operator/1, Relational Operator1/1
  Relational Operator1/1 -> Logical Operator/2
  Relational Operator/1 -> Logical Operator/1
  Logical Operator/1 -> Subsystem16/1(flag)
  Constant2/1 -> Relational Operator2/2
  SteerAngle/1 -> Abs/1
  Add3/1 -> Multiport Switch2/3
  Constant17/1 -> Add3/1
  Unit Delay2/1 -> Add3/2
  Constant22/1 -> Relational Operator19/2
  Multiport Switch2/1 -> Unit Delay2/1, Relational Operator19/1
  Constant18/1 -> Multiport Switch2/2
  Relational Operator2/1 -> Multiport Switch2/1
  Constant11/1 -> Relational Operator7/2
  TTC/1 -> Relational Operator7/1
  Relational Operator7/1 -> Subsystem1/1(flag)
  LatAccelLimit/1(Limit) -> Relational Operator5/2
  LatAccel/1 -> Relational Operator5/1
  Add2/1 -> Multiport Switch3/3
  Constant7/1 -> Add2/1
  Unit Delay3/1 -> Add2/2
  Constant8/1 -> Multiport Switch3/2
  Relational Operator5/1 -> Multiport Switch3/1
  Constant9/1 -> Relational Operator6/2
  Multiport Switch3/1 -> Unit Delay3/1, Relational Operator6/1
  Constant10/1 -> Relational Operator8/2
  LatDisLimit_C/1 -> Relational Operator8/1
  Add4/1 -> Multiport Switch4/3
  Constant12/1 -> Add4/1
  Unit Delay4/1 -> Add4/2
  Constant13/1 -> Multiport Switch4/2
  Relational Operator8/1 -> Multiport Switch4/1
  Constant14/1 -> Relational Operator9/2
  Multiport Switch4/1 -> Unit Delay4/1, Relational Operator9/1
  Relational Operator19/1 -> Subsystem2/1(flag)
  Relational Operator6/1 -> Subsystem4/1(flag)
  Relational Operator9/1 -> Subsystem5/1(flag)
  Subsystem1/1(maskCnst) -> Add7/2, Scope4/1
  Subsystem16/1(maskCnst) -> Add7/3, Scope1/1
  Subsystem2/1(maskCnst) -> Add7/4, Scope2/1
  Add7/1 -> Bitwise Operator/1
  Subsystem5/1(maskCnst) -> Add7/6, Scope5/1
  Subsystem4/1(maskCnst) -> Add7/5, Scope3/1
  Abs/1 -> Relational Operator2/1
  Constant19/1 -> Relational Operator12/2
  ESA_sts_Judge/1 -> Relational Operator12/1
  Relational Operator12/1 -> Subsystem6/1(flag)
  Subsystem6/1(maskCnst) -> Add7/1, Scope8/1

== system LACS/ESAsts/Allow2Steer ==
  LongiDis : Inport
  egoSpd : Inport  Port=2
  LatAcc : Inport  Port=3
  Dis_Need2Avoid : Inport  Port=4
  TTC : Inport  Port=5
  Add : Sum  Inputs=+-
  Add1 : Sum  Inputs=+-
  Add2 : Sum  Inputs=+-
  Constant : Constant  Value=0
  Constant1 : Constant  Value=LengthObj
  Constant11 : Constant  Value=TTCthreshold3
  Divide : Product  Inputs=*/
  Dot Product : DotProduct  InputSameDT=on  OutDataTypeStr=Inherit: Inherit via internal rule
  Dot Product1 : DotProduct  InputSameDT=on  OutDataTypeStr=Inherit: Inherit via internal rule
  Dot Product2 : DotProduct  InputSameDT=on  OutDataTypeStr=Inherit: Inherit via internal rule
  Gain : Gain  Gain=0.5
  Logical Operator4 : Logic  Inputs=3  AllPortsSameDT=off  OutDataTypeStr=boolean
  Relational Operator : RelationalOperator  Operator=<=  OutDataTypeStr=boolean  RndMeth=Simplest
  Relational Operator1 : RelationalOperator  OutDataTypeStr=boolean  RndMeth=Simplest
  Relational Operator7 : RelationalOperator  Operator=>  OutDataTypeStr=boolean  RndMeth=Simplest
  Scope{,1..5} (6 alike) : Scope
  Sqrt : Sqrt  SaturateOnIntegerOverflow=on
  Allow2Steer : Outport
  wires:
  egoSpd/1 -> Dot Product/2, Dot Product/1
  Dot Product/1 -> Divide/1
  LatAcc/1 -> Divide/2
  Divide/1 -> Add1/1, Dot Product1/2, Dot Product1/1
  Dot Product1/1 -> Add/1
  Dis_Need2Avoid/1 -> Add1/2
  Add1/1 -> Dot Product2/1, Dot Product2/2
  Dot Product2/1 -> Add/2
  Add/1 -> Scope5/1, Sqrt/1, Relational Operator/1
  Constant/1 -> Relational Operator/2
  Constant1/1 -> Gain/1
  LongiDis/1 -> Add2/1
  Gain/1 -> Add2/2
  Constant11/1 -> Relational Operator7/2
  TTC/1 -> Relational Operator7/1
  Sqrt/1 -> Scope4/1, Relational Operator1/2
  Add2/1 -> Scope3/1, Relational Operator1/1
  Relational Operator1/1 -> Scope2/1, Logical Operator4/1
  Relational Operator/1 -> Scope/1, Logical Operator4/2
  Relational Operator7/1 -> Scope1/1, Logical Operator4/3
  Logical Operator4/1 -> Allow2Steer/1

== system LACS/ESAsts/LatDisSafetyLimit1 ==
  te : Inport
  Abs : Abs
  Add : Sum  Inputs=+-
  Add1 : Sum
  Dis4MassPoint2RightAngle : Subsystem
  Dot Product : DotProduct  InputSameDT=on  OutDataTypeStr=Inherit: Inherit via internal rule
  Gain : Gain  Gain=0.5
  LatDisLimit_C : Outport
  wires:
  te/1 -> Gain/1
  [dx_r] -> Add/1
  Dis4MassPoint2RightAngle/1(r1) -> Add1/1
  Gain/1 -> Dot Product/1
  [vx_r] -> Dot Product/2
  Dot Product/1 -> Abs/1
  Abs/1 -> Add1/2
  Add1/1 -> Add/2
  Add/1 -> LatDisLimit_C/1
